simulink model "Motor_Controller"  (R2022a)
settings: Solver=FixedStepDiscrete  StartTime=0.0  StopTime=10.0  FixedStep=Tsi  RelTol=1e-3
values from neighbouring files (symbols this model uses):
  ID_MAP = -123.48613339558477 -123.48613339558477 -123.48613339558477 -123.48613339558477 -44.198759048598419 -53.055770135943519 -71.182249124603388 -83.754050470588808 -83.201735347031459 -88.439458490896953 -101.31743895897192 -109.70740328327217 -114.47442297164962 -116.44804085880824 -116.44444689073586 -115.21087408201925 -125.05741434421833 -119.17821915431119 -119.17821915431119 -119.17821915431119    [PMSM_plant_parameters.sldd]
  IQ_MAP = -339.52155191430609 -339.52155191430609 -339.52155191430609 -339.52155191430609 -298.63834091778995 -232.87622090578927 -192.99576989130705 -164.33367060179748 -138.47181888093323 -120.45650086696185 -110.27189121497848 -100.86088998300514 -91.979080238554033 -83.43921869931269 -75.095588141715126 -66.8406312898249 -66.136785837456742 -332.77622591535993 -332.77622591535993 -332.77622591535993 -33    [PMSM_plant_parameters.sldd]
  Ki_id = 710.3004    [ctrl_parameters.sldd]
  Ki_iq = 1061.5    [ctrl_parameters.sldd]
  Ki_omega = 200.0    [ctrl_parameters.sldd]
  Kp_id = 0.8779    [ctrl_parameters.sldd]
  Kp_iq = 1.0744    [ctrl_parameters.sldd]
  Kp_omega = 3.5    [ctrl_parameters.sldd]
  Ld = 0.00024368    [PMSM_plant_parameters.sldd]
  Lq = 0.00029758    [PMSM_plant_parameters.sldd]
  p = 8.0    [PMSM_plant_parameters.sldd]
  Pmax = 35000.0    [PMSM_plant_parameters.sldd]
  psim = 0.04366    [PMSM_plant_parameters.sldd]
  RPM_VECT = 0.0 500.0 1000.0 1500.0 2000.0 2500.0 3000.0 3500.0 4000.0 4500.0 5000.0 5500.0 6000.0 6500.0 7000.0 7500.0 8000.0    [PMSM_plant_parameters.sldd]
  Tmax = 205.0    [PMSM_plant_parameters.sldd]
  TQ_VECT = -205.0 -200.0 -195.0 -190.0 -185.0 -180.0 -175.0 -170.0 -165.0 -160.0 -155.0 -150.0 -145.0 -140.0 -135.0 -130.0 -125.0 -120.0 -115.0 -110.0 -105.0 -100.0 -95.0 -90.0 -85.0 -80.0 -75.0 -70.0 -65.0 -60.0 -55.0 -50.0 -45.0 -40.0 -35.0 -30.0 -25.0 -20.0 -15.0 -10.0 -5.0 0.0 5.0 10.0 15.0 20.0 25.0 30.0 35.0 40.0 45.0 50.0 55.0 60.0 65.0 70.0 75.0 80.0 85.0 90.0 95.0 100.0 105.0 110.0 115.0 120.0 125.0    [PMSM_plant_parameters.sldd]
  Tsi = 0.0001    [PMSM_system_data.sldd]
  Tso = 0.001    [PMSM_system_data.sldd]
  VDC_VECT = 275.0 300.0 325.0 350.0    [PMSM_plant_parameters.sldd]
  Vnom = 325.0    [PMSM_plant_parameters.sldd]
undefined symbols (not defined in the file or in its folder): denZC_id, denZC_iq, denZC_w, DiscIntNeverNeededParam, ee_sli_rtmsupport, gcbh, numZC_id, numZC_iq, numZC_w
libraries: simulink x8, eeTransforms x2
(part 2 of 2)

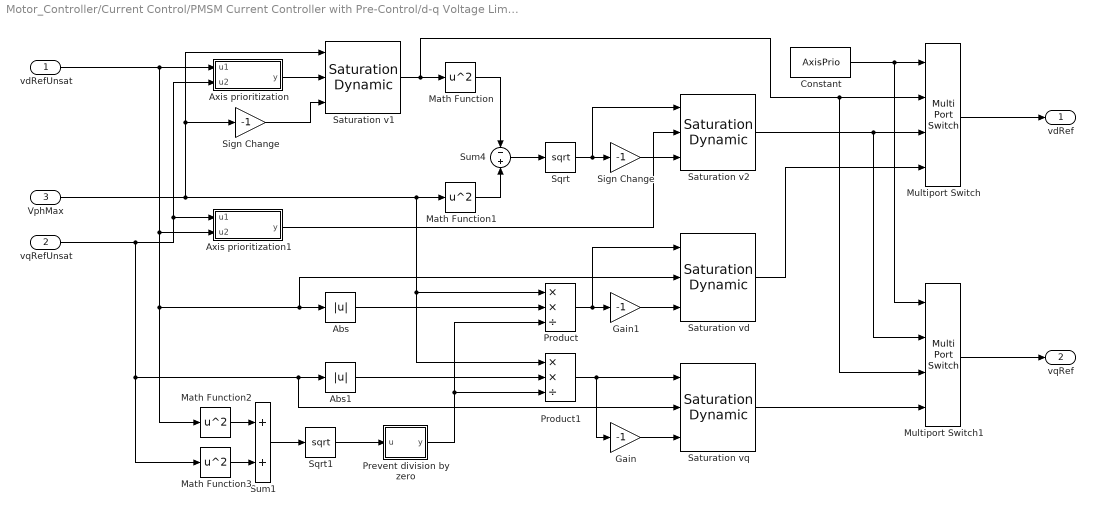
== system Motor_Controller/Current Control/PMSM Current Controller with Pre-Control/d-q Voltage Limiter ==
  vdRefUnsat : Inport  SampleTime=Ts
  vqRefUnsat : Inport  Port=2  SampleTime=Ts
  VphMax : Inport  Port=3  SampleTime=Ts
  Abs : Abs  SaturateOnIntegerOverflow=off
  Abs1 : Abs  SaturateOnIntegerOverflow=off
  Axis prioritization : Subsystem
  Axis prioritization1 : Subsystem
  Constant : Constant  Value=AxisPrio  OutDataTypeStr=single  SampleTime=Ts
  Gain : Gain  Gain=-1
  Gain1 : Gain  Gain=-1
  Math Function{,1..3} (4 alike) : Math  Operator=square  SignedPower=on
  Multiport Switch : MultiPortSwitch  SaturateOnIntegerOverflow=off  InputSameDT=off
  Multiport Switch1 : MultiPortSwitch  SaturateOnIntegerOverflow=off  InputSameDT=off
  Prevent division by zero : Subsystem
  Product : Product  Inputs=**/
  Product1 : Product  Inputs=**/
  Saturation v1 : simulink/Discontinuities/Saturation Dynamic  OutMin=[]  OutMax=[]  OutDataTypeStr=Inherit: Same as second input  OutDataType=fixdt(1, 16)  OutScaling=2^-10  DoSatur=off
  Saturation v2 : simulink/Discontinuities/Saturation Dynamic  OutMin=[]  OutMax=[]  OutDataTypeStr=Inherit: Same as second input  OutDataType=fixdt(1, 16)  OutScaling=2^-10  DoSatur=off
  Saturation vd : simulink/Discontinuities/Saturation Dynamic  OutMin=[]  OutMax=[]  OutDataTypeStr=Inherit: Same as second input  OutDataType=fixdt(1, 16)  OutScaling=2^-10  DoSatur=off
  Saturation vq : simulink/Discontinuities/Saturation Dynamic  OutMin=[]  OutMax=[]  OutDataTypeStr=Inherit: Same as second input  OutDataType=fixdt(1, 16)  OutScaling=2^-10  DoSatur=off
  Sign Change : Gain  Gain=-1
  "Sign Change " : Gain  Gain=-1
  Sqrt : Sqrt
  Sqrt1 : Sqrt
  Sum1 : Sum
  Sum4 : Sum  Inputs=-+
  vdRef : Outport  VectorParamsAs1DForOutWhenUnconnected=off
  vqRef : Outport  Port=2  VectorParamsAs1DForOutWhenUnconnected=off
  wires:
  "Sign Change "/1 -> Saturation v2/3
  Sqrt/1 -> "Sign Change "/1, Saturation v2/1
  Math Function/1 -> Sum4/1
  Sum4/1 -> Sqrt/1
  Math Function1/1 -> Sum4/2
  Sign Change/1 -> Saturation v1/3
  Saturation v1/1 -> Multiport Switch1/3, Multiport Switch/2, Math Function/1
  Axis prioritization1/1(y) -> Saturation v2/2
  Axis prioritization/1(y) -> Saturation v1/2
  vqRefUnsat/1 -> Saturation vq/2, Abs1/1, Math Function3/1, Axis prioritization1/1(u1), Axis prioritization/2(u2)
  Sum1/1 -> Sqrt1/1
  VphMax/1 -> Math Function1/1, Product1/1, Product/1, Saturation v1/1, Sign Change/1
  vdRefUnsat/1 -> Axis prioritization/1(u1), Math Function2/1, Saturation vd/2, Abs/1, Axis prioritization1/2(u2)
  Math Function2/1 -> Sum1/1
  Math Function3/1 -> Sum1/2
  Sqrt1/1 -> Prevent division by zero/1(u)
  Constant/1 -> Multiport Switch1/1, Multiport Switch/1
  Saturation v2/1 -> Multiport Switch/3, Multiport Switch1/2
  Multiport Switch/1 -> vdRef/1
  Multiport Switch1/1 -> vqRef/1
  Prevent division by zero/1(y) -> Product/3, Product1/3
  Abs/1 -> Product/2
  Abs1/1 -> Product1/2
  Product/1 -> Saturation vd/1, Gain1/1
  Product1/1 -> Saturation vq/1, Gain/1
  Saturation vq/1 -> Multiport Switch1/4
  Saturation vd/1 -> Multiport Switch/4
  Gain/1 -> Saturation vq/3
  Gain1/1 -> Saturation vd/3

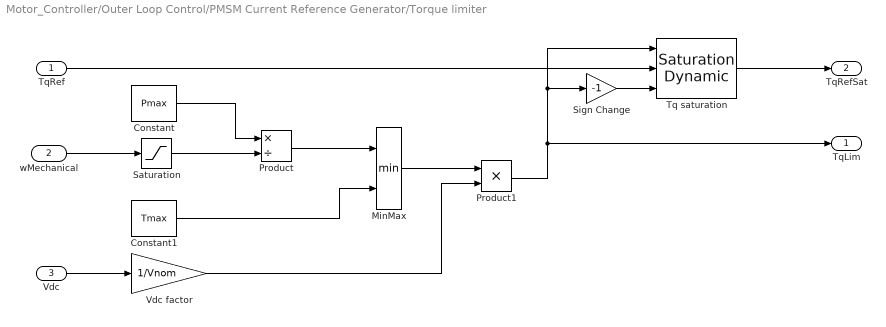
== system Motor_Controller/Outer Loop Control/PMSM Current Reference Generator/Torque limiter ==
  TqRef : Inport
  wMechanical : Inport  Port=2
  Vdc : Inport  Port=3
  Constant : Constant  Value=Pmax  OutDataTypeStr=single  SampleTime=Ts
  Constant1 : Constant  Value=Tmax  OutDataTypeStr=single  SampleTime=Ts
  MinMax : MinMax  Inputs=2
  Product : Product  Inputs=*/
  Product1 : Product
  Saturation : Saturate  UpperLimit=inf  LowerLimit=Pmax/Tmax
  Sign Change : Gain  Gain=-1
  Tq saturation : simulink/Discontinuities/Saturation Dynamic  OutMin=[]  OutMax=[]  OutDataTypeStr=Inherit: Same as second input  OutDataType=fixdt(1, 16)  OutScaling=2^-10  DoSatur=off
  Vdc factor : Gain  Gain=1/Vnom
  TqLim : Outport  VectorParamsAs1DForOutWhenUnconnected=off
  TqRefSat : Outport  Port=2  VectorParamsAs1DForOutWhenUnconnected=off
  wires:
  Tq saturation/1 -> TqRefSat/1
  Product1/1 -> Tq saturation/1, Sign Change/1, TqLim/1
  TqRef/1 -> Tq saturation/2
  Vdc/1 -> Vdc factor/1
  Constant1/1 -> MinMax/2
  wMechanical/1 -> Saturation/1
  Product/1 -> MinMax/1
  Constant/1 -> Product/1
  Saturation/1 -> Product/2
  Sign Change/1 -> Tq saturation/3
  MinMax/1 -> Product1/1
  Vdc factor/1 -> Product1/2

== system Motor_Controller/Outer Loop Control/Velocity Controller/Discrete PI Controller ==
  e : Inport  SampleTime=Ts
  du : Inport  Port=2  SampleTime=Ts
  Reset : Inport  Port=3  SampleTime=Ts
  Discrete-Time Integrator : DiscreteIntegrator  IntegratorMethod=Integration: Backward Euler  ExternalReset=rising  InitialCondition=x0  SampleTime=Ts  ICPrevOutput=DiscIntNeverNeededParam  ICPrevScaledInput=DiscIntNeverNeededParam
  Gain : Gain  Gain=Kp
  Gain1 : Gain  Gain=Ki
  Gain2 : Gain  Gain=Kaw
  Sum : Sum  Inputs=|++
  Sum1 : Sum  Inputs=|++
  Unit Delay : UnitDelay  SampleTime=Ts  HasFrameUpgradeWarning=on
  u : Outport  VectorParamsAs1DForOutWhenUnconnected=off
  wires:
  Unit Delay/1 -> Gain2/1
  Reset/1 -> Discrete-Time Integrator/2
  du/1 -> Unit Delay/1
  Sum1/1 -> Discrete-Time Integrator/1
  Gain2/1 -> Sum1/2
  e/1 -> Gain1/1, Gain/1
  Gain/1 -> Sum/1
  Gain1/1 -> Sum1/1
  Discrete-Time Integrator/1 -> Sum/2
  Sum/1 -> u/1

== system Motor_Controller/Current Control/PMSM Current Controller with Pre-Control/d-q Voltage Limiter/Axis prioritization ==
  u1 : Inport
  u2 : Inport  Port=2
  Compare To Constant : simulink/Logic and Bit Operations/Compare To Constant  relop===  const=1  OutDataTypeStr=boolean
  Constant : Constant  Value=AxisPrio  SampleTime=Ts
  Switch : Switch  Criteria=u2 ~= 0  Threshold=1  SaturateOnIntegerOverflow=off  InputSameDT=off
  y : Outport  VectorParamsAs1DForOutWhenUnconnected=off
  wires:
  u1/1 -> Switch/1
  u2/1 -> Switch/3
  Switch/1 -> y/1
  Constant/1 -> Compare To Constant/1
  Compare To Constant/1 -> Switch/2

== system Motor_Controller/Current Control/PMSM Current Controller with Pre-Control/d-q Voltage Limiter/Axis prioritization1 ==
  u1 : Inport
  u2 : Inport  Port=2
  Compare To Constant : simulink/Logic and Bit Operations/Compare To Constant  relop===  const=1  OutDataTypeStr=boolean
  Constant : Constant  Value=AxisPrio  SampleTime=Ts
  Switch : Switch  Criteria=u2 ~= 0  Threshold=1  SaturateOnIntegerOverflow=off  InputSameDT=off
  y : Outport  VectorParamsAs1DForOutWhenUnconnected=off
  wires:
  u1/1 -> Switch/1
  u2/1 -> Switch/3
  Switch/1 -> y/1
  Compare To Constant/1 -> Switch/2
  Constant/1 -> Compare To Constant/1

== system Motor_Controller/Current Control/PMSM Current Controller with Pre-Control/d-q Voltage Limiter/Prevent division by zero ==
  u : Inport
  Constant1 : Constant  Value=0.001
  Switch : Switch  Criteria=u2 > Threshold  Threshold=0.001  SaturateOnIntegerOverflow=off  InputSameDT=off
  y : Outport  VectorParamsAs1DForOutWhenUnconnected=off
  wires:
  Constant1/1 -> Switch/3
  u/1 -> Switch/1, Switch/2
  Switch/1 -> y/1
